simulink model "NlZkGeschlossenerKreis"  (Simulink 9.3)
settings: Solver=ode45  StartTime=0.0  StopTime=10.0  MaxStep=15e-3  RelTol=1e-3
values from neighbouring files (symbols this model uses):
  B_1 = 2.39e6    (= 2390000)    [A4Main.m]
  C_o = 36.5e6    (= 36500000)    [A4Main.m]
  C_p = 75e6    (= 75000000)    [A4Main.m]
  K_M = 1/63000    (= 1.5873015873e-05)    [A4Main.m]
  M_g = M_k + M_p    (= 268.7)    [A4Main.m]
  T_a = 0.015    [A4Main.m]
  U_step = 0.8    [A4Main.m]
undefined symbols (not defined in the file or in its folder): DiscIntNeverNeededParam
settings Model: Creator=wredi  LastModifiedBy=wredi
settings DataIOCC: SaveFormat=Dataset  SignalLoggingSaveFormat=Dataset  ReturnWorkspaceOutputs=on
settings DebuggingCC: UnderspecifiedInitializationDetection=Simplified  MergeDetectMultiDrivingBlocksExec=error  FcnCallInpInsideContextMsg=error  SFUnexpectedBacktrackingDiag=error  SFNoUnconditionalDefaultTransitionDiag=error  SFExecutionAtInitializationDiag=warning
settings HardwareCC: ProdBitPerPointer=64  ProdBitPerSizeT=64  ProdBitPerPtrDiffT=64  ProdLargestAtomicFloat=Float  ProdIntDivRoundTo=Zero  ProdEndianess=LittleEndian  ProdWordSize=64  ProdHWDeviceType=Intel->x86-64 (Windows64)
settings ModelReferenceCC: PropagateSignalLabelsOutOfModel=on
settings SFSimCC: SimUseLocalCustomCode=on
settings RTWCC: RTWUseLocalCustomCode=on
settings CodeAppCC: StateflowObjectComments=off
settings GRTTargetCC: TargetLangStandard=C99 (ISO)  CombineOutputUpdateFcns=on  GRTInterface=off
settings ConfigComp: CovMetricSettings=dwe  CovHtmlReporting=off  CovSaveCumulativeToWorkspaceVar=off  CovSaveSingleToWorkspaceVar=off  CovExternalEMLEnable=on

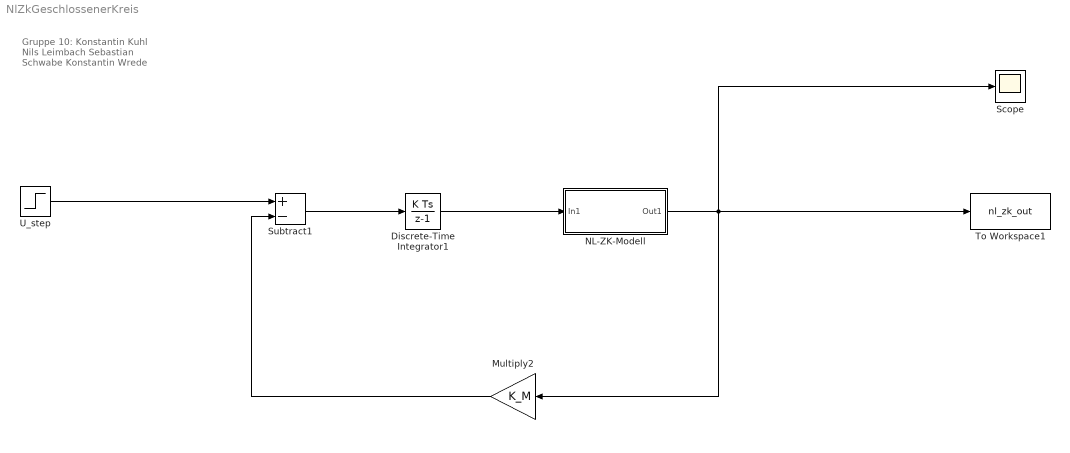
== system NlZkGeschlossenerKreis ==
  note: Gruppe 10:
      | Konstantin Kuhl
      | Nils Leimbach
      | Sebastian Schwabe
      | Konstantin Wrede
  Discrete-Time Integrator1 : DiscreteIntegrator  gainval=K_I_controller  SampleTime=T_a  ICPrevOutput=DiscIntNeverNeededParam  ICPrevScaledInput=DiscIntNeverNeededParam
  Multiply2 : Gain  Gain=K_M
  NL-ZK-Modell : Subsystem
  Scope : Scope
  Subtract1 : Sum  Inputs=+-
  To Workspace1 : ToWorkspace  VariableName=nl_zk_out  SaveFormat=Structure With Time  SampleTime=-1
  U_step : Step  After=U_step  SampleTime=0
  wires:
  U_step/1 -> Subtract1/1
  Multiply2/1 -> Subtract1/2
  NL-ZK-Modell/1(Out1) -> Scope/1, To Workspace1/1, Multiply2/1
  Discrete-Time Integrator1/1 -> NL-ZK-Modell/1(In1)
  Subtract1/1 -> Discrete-Time Integrator1/1

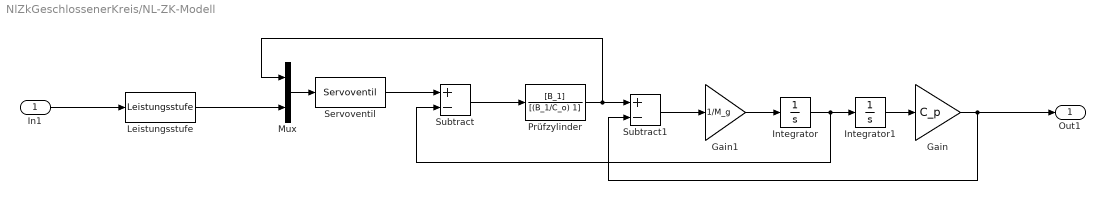
== system NlZkGeschlossenerKreis/NL-ZK-Modell ==
  In1 : Inport
  Gain : Gain  Gain=C_p
  Gain1 : Gain  Gain=1/M_g
  Integrator : Integrator
  Integrator1 : Integrator
  Leistungsstufe : MATLABFcn  MATLABFcn=Leistungsstufe  OutputDimensions=1
  Mux : Mux  Inputs=2
  Prüfzylinder : TransferFcn  Numerator=[B_1]  Denominator=[(B_1/C_o) 1]
  "Servoventil " : MATLABFcn  MATLABFcn=Servoventil  OutputDimensions=1  Output1D=off
  Subtract : Sum  Inputs=+-
  Subtract1 : Sum  Inputs=+-
  Out1 : Outport
  wires:
  In1/1 -> Leistungsstufe/1
  Integrator/1 -> Subtract/2, Integrator1/1
  Gain1/1 -> Integrator/1
  Prüfzylinder/1 -> Mux/1, Subtract1/1
  "Servoventil "/1 -> Subtract/1
  Subtract/1 -> Prüfzylinder/1
  Subtract1/1 -> Gain1/1
  Gain/1 -> Out1/1, Subtract1/2
  Integrator1/1 -> Gain/1
  Leistungsstufe/1 -> Mux/2
  Mux/1 -> "Servoventil "/1
